simulink model "Chap9_5"  (Simulink 3.00)
settings: Solver=ode45  StartTime=0  StopTime=5  RelTol=1e-3
values from neighbouring files (symbols this model uses):
  b = 1    [Chap9_5i.m]    (also in chap9_7i.m = 0.5)
  bc = 30.0    (= 30)    [Chap9_5i.m]    (also in chap9_6i.m = 3)
  bc1 = bc/Gain    (= 0.454545454545)    [Chap9_5i.m]
  Ce = 0.001    [Chap9_5i.m]    (also in chap9_3.m = 1.2; chap9_4plant.m = 1.2; chap9_6i.m)
  Fc = 15    [CHAP9_3F.M]    (also in Chap9_5i.m = 100; chap9_1eq.m = 0.28; chap9_2s.m = 0.28; chap9_4plant.m)
  Fc1 = Fc/Gain    (= 1.51515151515)    [Chap9_5i.m]
  J = 2    [Chap9_5i.m]    (also in chap9_1eq.m = 1; chap9_2i.m = 1; chap9_3.m = 0.6; chap9_4plant.m = 0.6)
  kd = 6    [Chap9_5i.m]    (also in chap9_6i.m; chap9_7i.m)
  kdd = 1.5    [Chap9_5i.m]    (also in chap9_6i.m = 5)
  ki = 0.001    [Chap9_5i.m]    (also in chap9_6i.m)
  kii = 0.1    [Chap9_5i.m]    (also in chap9_6i.m = 1)
  km = 1.0    (= 1)    [Chap9_5i.m]    (also in chap9_6i.m = 10)
  kpp = 150    [Chap9_5i.m]    (also in chap9_6i.m = 8)
  ku = 11    [Chap9_5i.m]    (also in chap9_6i.m)
  kv = 2.0    (= 2)    [CHAP9_3F.M]    (also in Chap9_5i.m; chap9_4plant.m; chap9_6i.m; chap9_7i.m)
  L = 0.001    [Chap9_5i.m]    (also in chap9_6i.m)
  R = 1    [Chap9_5i.m]    (also in chap9_3.m = 7.77; chap9_4plant.m = 7.77; chap9_6i.m)
undefined symbols (not defined in the file or in its folder): sgn
libraries: simulink_extras x1

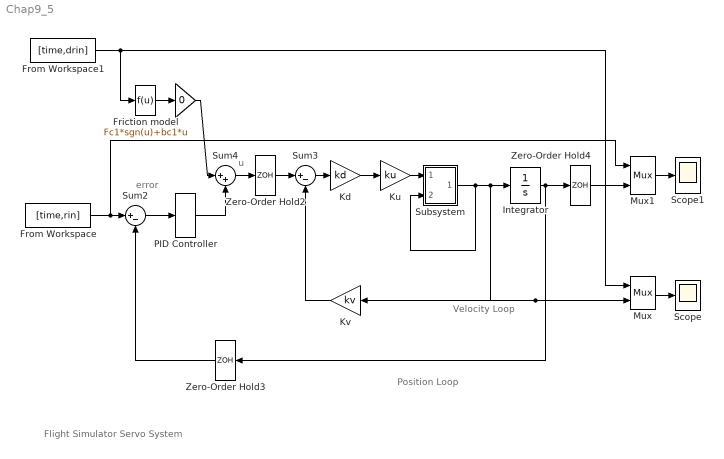
== system Chap9_5 ==
  note: u
  note: Position Loop
  note: Velocity Loop
  note: Flight Simulator Servo System
  note: error
  "     " : Gain  Gain=0  SaturateOnIntegerOverflow=on
  Friction model : Fcn  Expr=Fc1*sgn(u)+bc1*u
  From Workspace : FromWorkspace  VariableName=[time,rin]  SampleTime=0.001  HoldFinalValue=off
  From Workspace1 : FromWorkspace  VariableName=[time,drin]  SampleTime=0.001  HoldFinalValue=off
  Integrator : Integrator  ExternalReset=none  InitialConditionSource=internal  InitialCondition=0  LimitOutput=off  UpperSaturationLimit=inf  LowerSaturationLimit=-inf  ShowSaturationPort=off  ShowStatePort=off  AbsoluteTolerance=auto
  Kd : Gain  Gain=kd  SaturateOnIntegerOverflow=on
  Ku : Gain  Gain=ku  SaturateOnIntegerOverflow=on
  Kv : Gain  Orientation=left  Gain=kv  SaturateOnIntegerOverflow=on
  Mux : Mux  Inputs=2
      settings: DisplayOption=none
  Mux1 : Mux  Inputs=2
      settings: DisplayOption=none
  PID Controller : simulink_extras/Additional Linear/PID Controller  P=kpp  I=kii  D=kdd
  Scope : Scope
      settings: TimeRange=auto  YMin=-7  YMax=7  SaveToWorkspace=off  SaveName=ScopeData  MaxRows=50000
  Scope1 : Scope
      settings: TimeRange=auto  YMin=-1.73472e-018  YMax=0.019  SaveToWorkspace=off  SaveName=ScopeData  MaxRows=50000
  Subsystem : Subsystem
  Sum2 : Sum  Inputs=|+-  SaturateOnIntegerOverflow=on
  Sum3 : Sum  Inputs=|+-  SaturateOnIntegerOverflow=on
  Sum4 : Sum  Inputs=|++  SaturateOnIntegerOverflow=on
  Zero-Order Hold2 : ZeroOrderHold  SampleTime=0.001
  Zero-Order Hold3 : ZeroOrderHold  Orientation=left  SampleTime=0.001
  Zero-Order Hold4 : ZeroOrderHold  SampleTime=0.001
  wires:
  Sum3/1 -> Kd/1
  Mux/1 -> Scope/1
  Mux1/1 -> Scope1/1
  Subsystem/1(Out1) -> Integrator/1, Kv/1, Mux/2, Subsystem/2(In2)
  Zero-Order Hold4/1 -> Mux1/2
  Integrator/1 -> Zero-Order Hold3/1, Zero-Order Hold4/1
  Sum2/1 -> PID Controller/1
  Zero-Order Hold3/1 -> Sum2/2
  From Workspace1/1 -> Mux/1, Friction model/1
  Friction model/1 -> "     "/1
  "     "/1 -> Sum4/1
  Kv/1 -> Sum3/2
  PID Controller/1 -> Sum4/2
  Sum4/1 -> Zero-Order Hold2/1
  Ku/1 -> Subsystem/1(In1)
  Kd/1 -> Ku/1
  From Workspace/1 -> Mux1/1, Sum2/1
  Zero-Order Hold2/1 -> Sum3/1

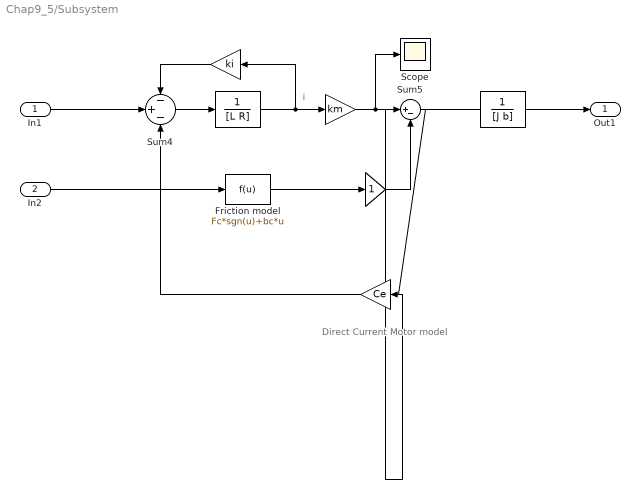
== system Chap9_5/Subsystem ==
  note: i
  note: Direct Current Motor model
  In1 : Inport  Port=1  PortWidth=-1  SampleTime=-1  DataType=auto
      settings: SignalType=auto
  In2 : Inport  Port=2  PortWidth=-1  SampleTime=-1  DataType=auto
      settings: SignalType=auto
  "    " : Gain  Orientation=left  Gain=Ce  SaturateOnIntegerOverflow=on
  "      " : Gain  Orientation=left  Gain=ki  SaturateOnIntegerOverflow=on
  "  " : Gain  Gain=km  SaturateOnIntegerOverflow=on
  "   " : TransferFcn  Numerator=[1]  Denominator=[L R]
  "    " : TransferFcn  Numerator=[1]  Denominator=[J b]
  "     " : Gain  Gain=1  SaturateOnIntegerOverflow=on
  Friction model : Fcn  Expr=Fc*sgn(u)+bc*u
  Scope : Scope
      settings: TimeRange=auto  YMin=-80  YMax=80  SaveToWorkspace=off  SaveName=ScopeData  MaxRows=50000
  Sum4 : Sum  Inputs=-+-  SaturateOnIntegerOverflow=off
  Sum5 : Sum  Inputs=|+-  SaturateOnIntegerOverflow=on
  Out1 : Outport  Port=1
  wires:
  Sum5/1 -> "    "/1
  "    "/1 -> Sum4/3
  "    "/1 -> "    "/1, Out1/1
  "   "/1 -> "      "/1, "  "/1
  "      "/1 -> Sum4/1
  "  "/1 -> Sum5/1, Scope/1
  "     "/1 -> Sum5/2
  Friction model/1 -> "     "/1
  In1/1 -> Sum4/2
  In2/1 -> Friction model/1
  Sum4/1 -> "   "/1
